simulink model "liqlevel"  (R2017a)
settings: Solver=ode45  StartTime=0.0  StopTime=(length(uin)-1)*Ts  RelTol=1e-3  EnableMultiTasking=on
model workspace (MATLAB code in the model file):
  | Cv = 1.5; Ac = 2;
  | x0 = 9;
  | uss = Cv*sqrt(x0);
  | 
  | tau = Ac*2*sqrt(x0)/Cv;
  | sampfact =2;
  | Ts = tau/sampfact;
  | f_max = (4/sampfact)/(2*pi);
  | B_max = 1/5;
  | 
  | usig = idinput(255,'prbs',[0 B_max],[-1 1]);
  | uin = [(0:1:length(usig)-1)'*Ts (usig*0.05+1)*uss];
settings Model: ExtModeAutoUpdateStatusClock=off  OrderedModelArguments=off  Creator=arun  LastModifiedBy=Ramziyya
settings DataIOCC: SaveFormat=Array  SignalLoggingSaveFormat=ModelDataLogs  SaveState=on
settings OptimizationCC: ExpressionDepthLimit=2147483647  InitFltsAndDblsToZero=on  LifeSpan=inf
settings DebuggingCC: SaveWithParameterizedLinksMsg=none  UnderspecifiedInitializationDetection=Classic  MergeDetectMultiDrivingBlocksExec=none  SolverPrmCheckMsg=warning  FcnCallInpInsideContextMsg=warning  StateNameClashWarn=warning  SFUnexpectedBacktrackingDiag=warning  SFNoUnconditionalDefaultTransitionDiag=warning  SFExecutionAtInitializationDiag=none
settings HardwareCC: ProdBitPerPointer=32  ProdBitPerSizeT=32  ProdBitPerPtrDiffT=32  ProdLargestAtomicFloat=None  ProdIntDivRoundTo=Undefined  ProdEndianess=Unspecified  ProdWordSize=32  ProdHWDeviceType=32-bit Generic
settings ModelReferenceCC: PropagateSignalLabelsOutOfModel=off
settings GRTTargetCC: TargetFcnLib=ansi_tfl_tmw.mat  TargetLangStandard=C89/C90 (ANSI)  GeneratePreprocessorConditionals=Disable all  CombineOutputUpdateFcns=off  GRTInterface=on
settings ConfigComp: CovMetricSettings=dw  CovHtmlReporting=on  CovSaveCumulativeToWorkspaceVar=on  CovSaveSingleToWorkspaceVar=on  CovExternalEMLEnable=off  CovSFcnEnable=off

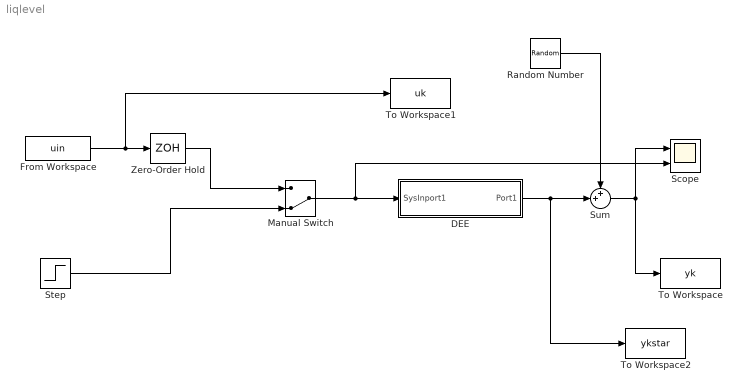
== system liqlevel ==
  DEE : Subsystem  mask(Differential Equation Editor (DEE)){}
      settings: OpenFcn=diffeqed
      mask Display: disp('Differential Equation\n Editor')
  From Workspace : FromWorkspace  VariableName=uin  SampleTime=Ts  Interpolate=off  OutputAfterFinalValue=Holding final value
  Manual Switch : ManualSwitch  CurrentSetting=0
  Random Number : RandomNumber  Variance=0.5  SampleTime=Ts
  Scope : Scope  NumInputPorts=2
  Step : Step  After=4.5  SampleTime=1
  Sum : Sum  Inputs=++|
  To Workspace : ToWorkspace  VariableName=yk  SampleTime=Ts
  To Workspace1 : ToWorkspace  VariableName=uk  SampleTime=Ts
  To Workspace2 : ToWorkspace  VariableName=ykstar  SampleTime=Ts
  Zero-Order Hold : ZeroOrderHold  SampleTime=Ts
  wires:
  Manual Switch/1 -> DEE/1(SysInport1), Scope/2
  From Workspace/1 -> Zero-Order Hold/1, To Workspace1/1
  Step/1 -> Manual Switch/2
  Zero-Order Hold/1 -> Manual Switch/1
  DEE/1(Port1) -> Sum/2, To Workspace2/1
  Random Number/1 -> Sum/1
  Sum/1 -> Scope/1, To Workspace/1

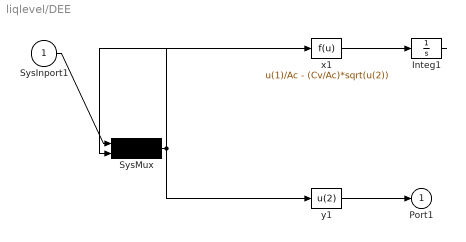
== system liqlevel/DEE ==
  SysInport1 : Inport
  Integ1 : Integrator  InitialCondition=x0
  SysMux : Mux  Inputs=2
  x1 : Fcn  Expr=u(1)/Ac - (Cv/Ac)*sqrt(u(2))
  y1 : Fcn  Expr=u(2)
  Port1 : Outport
  wires:
  SysInport1/1 -> SysMux/1
  SysMux/1 -> x1/1, y1/1
  x1/1 -> Integ1/1
  Integ1/1 -> SysMux/2
  y1/1 -> Port1/1
